simulink model "pmsm_model_2021_06_21"  (R2020a)
settings: Solver=ode23tb  StartTime=0.0  StopTime=simlength
values from neighbouring files (symbols this model uses):
  Jm = 1    [init_pmsm_2021_06_21.m]
  Ts = 1/10e3    (= 0.0001)    [init_pmsm_2021_06_21.m]
libraries: fl_lib x10, nesl_utility x9, flexshaft_lib x1, pmsm_uvw_lib x1
settings Model: SimulationMode=accelerator  Creator=dbagn  LastModifiedBy=dabagnara
settings SolverCC: ZeroCrossControl=DisableAll  SolverResetMethod=Robust
settings DataIOCC: ReturnWorkspaceOutputs=off

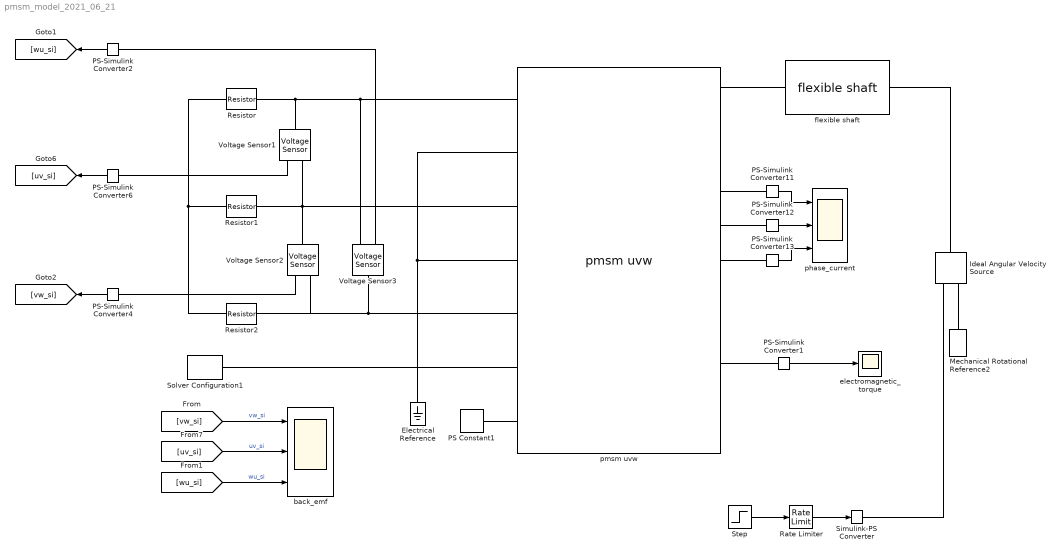
== system pmsm_model_2021_06_21 ==
  Electrical Reference : fl_lib/Electrical/Electrical Elements/Electrical Reference
  Ideal Angular Velocity Source : fl_lib/Mechanical/Mechanical Sources/Ideal Angular Velocity Source
  Mechanical Rotational Reference2 : fl_lib/Mechanical/Rotational Elements/Mechanical Rotational Reference
  PS Constant1 : fl_lib/Physical Signals/Sources/PS Constant  constant=psi_m V*s
  PS-Simulink Converter1 : nesl_utility/PS-Simulink Converter  PhysicalDomain=network_engine_domain  SubClassName=ps_output  LeftPortType=input  RightPortType=output  PseudoPeriodic=off  Frequencies=[]  Unit=N*m  AffineConversion=on
  PS-Simulink Converter11 : nesl_utility/PS-Simulink Converter  PhysicalDomain=network_engine_domain  SubClassName=ps_output  LeftPortType=input  RightPortType=output  PseudoPeriodic=off  Frequencies=[]  Unit=A  AffineConversion=on
  PS-Simulink Converter12 : nesl_utility/PS-Simulink Converter  PhysicalDomain=network_engine_domain  SubClassName=ps_output  LeftPortType=input  RightPortType=output  PseudoPeriodic=off  Frequencies=[]  Unit=A  AffineConversion=on
  PS-Simulink Converter13 : nesl_utility/PS-Simulink Converter  PhysicalDomain=network_engine_domain  SubClassName=ps_output  LeftPortType=input  RightPortType=output  PseudoPeriodic=off  Frequencies=[]  Unit=A  AffineConversion=on
  PS-Simulink Converter2 : nesl_utility/PS-Simulink Converter  PhysicalDomain=network_engine_domain  SubClassName=ps_output  LeftPortType=input  RightPortType=output  PseudoPeriodic=off  Frequencies=[]  Unit=1  AffineConversion=off
  PS-Simulink Converter4 : nesl_utility/PS-Simulink Converter  PhysicalDomain=network_engine_domain  SubClassName=ps_output  LeftPortType=input  RightPortType=output  PseudoPeriodic=off  Frequencies=[]  Unit=1  AffineConversion=off
  PS-Simulink Converter6 : nesl_utility/PS-Simulink Converter  PhysicalDomain=network_engine_domain  SubClassName=ps_output  LeftPortType=input  RightPortType=output  PseudoPeriodic=off  Frequencies=[]  Unit=1  AffineConversion=off
  Rate Limiter : RateLimiter  RisingSlewLimit=3100  FallingSlewLimit=-3100  SampleTimeMode=inherited
  Resistor : fl_lib/Electrical/Electrical Elements/Resistor  R=1 Ohm  i_specify=off  i_priority=None  i=0 A  i_nominal_specify=off  i_nominal_unit=A  i_nominal_value=1  v_specify=off  v_priority=None  v=0 V  v_nominal_specify=off  v_nominal_unit=V  v_nominal_value=1
  Resistor1 : fl_lib/Electrical/Electrical Elements/Resistor  R=1 Ohm  i_specify=off  i_priority=None  i=0 A  i_nominal_specify=off  i_nominal_unit=A  i_nominal_value=1  v_specify=off  v_priority=None  v=0 V  v_nominal_specify=off  v_nominal_unit=V  v_nominal_value=1
  Resistor2 : fl_lib/Electrical/Electrical Elements/Resistor  R=1 Ohm  i_specify=off  i_priority=None  i=0 A  i_nominal_specify=off  i_nominal_unit=A  i_nominal_value=1  v_specify=off  v_priority=None  v=0 V  v_nominal_specify=off  v_nominal_unit=V  v_nominal_value=1
  Simulink-PS Converter : nesl_utility/Simulink-PS Converter  PhysicalDomain=network_engine_domain  SubClassName=ps_input  LeftPortType=input  RightPortType=output  PseudoPeriodic=off  Frequencies=[]  NoiseDistribution=none  NoiseParameters=[]  Unit=rpm  AffineConversion=on  FilteringAndDerivatives=provide  SimscapeFilterOrder=1  InputFilterTimeConstant=0.001  UdotUserProvided=0
  Solver Configuration1 : nesl_utility/Solver Configuration  PhysicalDomain=network_engine_domain  SubClassName=solver  LeftPortType=input  RightPortType=generic  Tones=[]  Harmonics=[]  SimulateNoise=off  Profile=off  UseLocalSampling=off  EnableSwitchedLinearOptims=on  FrequencyDomain=off  UseCCode=off  RelTol=0.001  AbsTol=1e-06  MinStep=1e-09  ToWorkspace=off  RevertToSquareIcSolve=off  NumHomotopyIterations=100  PhasorMode=off  PhasorModeNumHarmonics=1  DoDC=off  ResidualTolerance=1e-09  UseLocalSolver=on  LocalSolverChoice=NE_BACKWARD_EULER_ADVANCER  LocalSolverSampleTime=Ts/10  DoFixedCost=on  MaxNonlinIter=3  MaxModeIter=2  LinearAlgebra=auto  EquationFormulation=NE_TIME_EF  DelaysMemoryBudget=1024*4  AutomaticFiltering=on  FilteringTimeConstant=Ts  PartitionStorageMethod=AS_NEEDED  PartitionMemoryBudget=1024  PartitionMethod=ROBUST
  Step : Step  After=3100  SampleTime=0
  Voltage Sensor1 : fl_lib/Electrical/Electrical Sensors/Voltage Sensor
  Voltage Sensor2 : fl_lib/Electrical/Electrical Sensors/Voltage Sensor
  Voltage Sensor3 : fl_lib/Electrical/Electrical Sensors/Voltage Sensor
  back_emf : Scope  NumInputPorts=3
  electromagnetic_torque : Scope
  flexible shaft : flexshaft_lib/flexible shaft  b1=0 N*m/(rad/s)  J1=0.125 kg*m^2  b2=0 N*m/(rad/s)  J2=0.125 kg*m^2  b_theta=1 N*m/(rad/s)  k_theta=1e5 N*m/rad  w_1_specify=off  w_1_priority=None  w_1=0 rad/s  w_1_nominal_specify=off  w_1_nominal_unit=rad/s  w_1_nominal_value=1  w_2_specify=off  w_2_priority=None  w_2=0 rad/s  w_2_nominal_specify=off  w_2_nominal_unit=rad/s  w_2_nominal_value=1  t_1_specify=off  t_1_priority=None  t_1=0 N*m  t_1_nominal_specify=off  t_1_nominal_unit=N*m  t_1_nominal_value=1  t_2_specify=off  t_2_priority=None  t_2=0 N*m  t_2_nominal_specify=off  t_2_nominal_unit=N*m  t_2_nominal_value=1  t_theta_specify=off  t_theta_priority=None  t_theta=0 N*m  t_theta_nominal_specify=off  t_theta_nominal_unit=N*m  t_theta_nominal_value=1
      settings: InternalSimscapePortConfiguration="{\"Bottom\":[],\"Left\":[{\"id\":\"S1\",\"label\":\"S1\",\"type\":\"foundation.mechanical.rotational.rotational\"}],\"Right\":[{\"id\":\"S2\",\"label\":\"S2\",\"type\":\"foundation.mechanical.rotational.rotational\"}],\"Top\":[]}"
  phase_current : Scope  NumInputPorts=3
  pmsm uvw : pmsm_uvw_lib/pmsm uvw  number_poles=number_poles  psi_M=psi_m s*V  Lmu=Lmu H  Ls=Ls H  Lb=Lb H  Rs=Rs Ohm  J=Jm kg*m^2  b=0 N*m/(rad/s)  omega_specify=off  omega_priority=None  omega=0 rad/s  omega_nominal_specify=off  omega_nominal_unit=rad/s  omega_nominal_value=1  theta_specify=off  theta_priority=None  theta=0 rad  theta_nominal_specify=off  theta_nominal_unit=rad  theta_nominal_value=1  iu_specify=off  iu_priority=None  iu=0 A  iu_nominal_specify=off  iu_nominal_unit=A  iu_nominal_value=1  iv_specify=off  iv_priority=None  iv=0 A  iv_nominal_specify=off  iv_nominal_unit=A  iv_nominal_value=1  iw_specify=off  iw_priority=None  iw=0 A  iw_nominal_specify=off  iw_nominal_unit=A  iw_nominal_value=1  id_specify=off  id_priority=None  id=0 A  id_nominal_specify=off  id_nominal_unit=A  id_nominal_value=1  iq_specify=off  iq_priority=None  iq=0 A  iq_nominal_specify=off  iq_nominal_unit=A  iq_nominal_value=1  uv_specify=off  uv_priority=None  uv=0 V  uv_nominal_specify=off  uv_nominal_unit=V  uv_nominal_value=1  uu_specify=off  uu_priority=None  uu=0 V  uu_nominal_specify=off  uu_nominal_unit=V  uu_nominal_value=1  uw_specify=off  uw_priority=None  uw=0 V  uw_nominal_specify=off  uw_nominal_unit=V  uw_nominal_value=1  phi_u_specify=off  phi_u_priority=High  phi_u=1 s*V  phi_u_nominal_specify=off  phi_u_nominal_unit=s*V  phi_u_nominal_value=1  phi_v_specify=off  phi_v_priority=None  phi_v=0 s*V  phi_v_nominal_specify=off  phi_v_nominal_unit=s*V  phi_v_nominal_value=1  phi_w_specify=off  phi_w_priority=None  phi_w=0 s*V  phi_w_nominal_specify=off  phi_w_nominal_unit=s*V  phi_w_nominal_value=1  phi_d_specify=off  phi_d_priority=None  phi_d=0 s*V  phi_d_nominal_specify=off  phi_d_nominal_unit=s*V  phi_d_nominal_value=1  phi_q_specify=off  phi_q_priority=None  phi_q=0 s*V  phi_q_nominal_specify=off  phi_q_nominal_unit=s*V  phi_q_nominal_value=1  psi_d_specify=off  psi_d_priority=None  psi_d=0 s*V  psi_d_nominal_specify=off  psi_d_nominal_unit=s*V  psi_d_nominal_value=1  psi_q_specify=off  psi_q_priority=None  psi_q=0 s*V  psi_q_nominal_specify=off  psi_q_nominal_unit=s*V  psi_q_nominal_value=1  tau_l_specify=off  tau_l_priority=None  tau_l=0 N*m  tau_l_nominal_specify=off  tau_l_nominal_unit=N*m  tau_l_nominal_value=1  tau_m_specify=off  tau_m_priority=None  tau_m=0 N*m  tau_m_nominal_specify=off  tau_m_nominal_unit=N*m  tau_m_nominal_value=1
      settings: InternalSimscapePortConfiguration="{\"Bottom\":[],\"Left\":[{\"id\":\"uu_p\",\"label\":\"_uu+_\",\"type\":\"foundation.electrical.electrical\"},{\"id\":\"uu_n\",\"label\":\"_uu-_\",\"type\":\"foundation.electrical.electrical\"},{\"id\":\"uv_p\",\"label\":\"_uv+_\",\"type\":\"foundation.electrical.electrical\"},{\"id\":\"uv_n\",\"label\":\"_uv-_\",\"type\":\"foundation.electrical.electrical\"},{\"id\":\"uw_p\",\"label\":\"_uw+_\",\"type\":\"foundation.electrical.electrical\"},{\"id\":\"uw_n\",\"label\":\"_uw-_\",\"type\":\"foundation.electrical.electrical\"},{\"id\":\"psi_m\",\"label\":\"_psi_m_\",\"type\":\"input\"}],\"Right\":[{\"id\":\"S\",\"label\":\"_S_\",\"type\":\"foundation.mechanical.rotational.rotational\"},{\"id\":\"id_out\",\"label\":\"_id_\",\"type\":\"output\"},{\"id\":\"iq_out\",\"label\":\"_iq_\",\"type\":\"output\"},{\"id\":\"iu_out\",\"label\":\"_iu_\",\"type\":\"output\"},{\"id\":\"iv_out\",\"label\":\"_iv_\",\"type\":\"output\"},{\"id\":\"iw_out\",\"label\":\"_iw_\",\"type\":\"output\"},{\"id\":\"phi_d_out\",\"label\":\"_phi_d_\",\"type\":\"output\"},{\"id\":\"phi_q_out\",\"label\":\"_phi_q\",\"type\":\"output\"},{\"id\":\"tau_out\",\"label\":\"_torque_\",\"type\":\"output\"},{\"id\":\"omega_out\",\"label\":\"_omega_elec_\",\"type\":\"output\"},{\"id\":\"theta_out\",\"label\":\"_theta_elec_\",\"type\":\"output\"}],\"Top\":[]}"
  wires:
  [uv_si] -> back_emf/2  "uv_si"
  PS-Simulink Converter1/1 -> electromagnetic_torque/1
  PS-Simulink Converter4/1 -> [vw_si]
  PS-Simulink Converter6/1 -> [uv_si]
  [vw_si] -> back_emf/1  "vw_si"
  PS-Simulink Converter2/1 -> [wu_si]
  [wu_si] -> back_emf/3  "wu_si"
  PS-Simulink Converter12/1 -> phase_current/2
  PS-Simulink Converter11/1 -> phase_current/1
  PS-Simulink Converter13/1 -> phase_current/3
  Step/1 -> Rate Limiter/1
  Rate Limiter/1 -> Simulink-PS Converter/1
  connections:
  Voltage Sensor1/RConn2 -- Resistor1/RConn1 -- Voltage Sensor2/LConn1 -- pmsm uvw/LConn3
  Resistor/LConn1 -- Resistor1/LConn1 -- Resistor2/LConn1
  pmsm uvw/LConn2 -- pmsm uvw/LConn4 -- pmsm uvw/LConn6 -- Electrical Reference/LConn1 -- Solver Configuration1/RConn1
  Resistor2/RConn1 -- Voltage Sensor2/RConn2 -- Voltage Sensor3/LConn1 -- pmsm uvw/LConn5
  Voltage Sensor1/LConn1 -- Voltage Sensor3/RConn2 -- pmsm uvw/LConn1 -- Resistor/RConn1
  Mechanical Rotational Reference2/LConn1 -- Ideal Angular Velocity Source/RConn2
  pmsm uvw/RConn9 -- PS-Simulink Converter1/LConn1
  Voltage Sensor1/RConn1 -- PS-Simulink Converter6/LConn1
  PS-Simulink Converter4/LConn1 -- Voltage Sensor2/RConn1
  PS-Simulink Converter2/LConn1 -- Voltage Sensor3/RConn1
  PS Constant1/RConn1 -- pmsm uvw/LConn7
  Ideal Angular Velocity Source/LConn1 -- flexible shaft/RConn1
  flexible shaft/LConn1 -- pmsm uvw/RConn1
  pmsm uvw/RConn6 -- PS-Simulink Converter13/LConn1
  pmsm uvw/RConn4 -- PS-Simulink Converter11/LConn1
  pmsm uvw/RConn5 -- PS-Simulink Converter12/LConn1
  Simulink-PS Converter/RConn1 -- Ideal Angular Velocity Source/RConn1
